simulink model "simulink_p"  (R2018b)
settings: Solver=VariableStepAuto  StartTime=0.0  StopTime=10.0  RelTol=1e-3
undefined symbols (not defined in the file): kp, kp1, td, ti, ti1
settings Model: Creator=tiago  LastModifiedBy=tiago

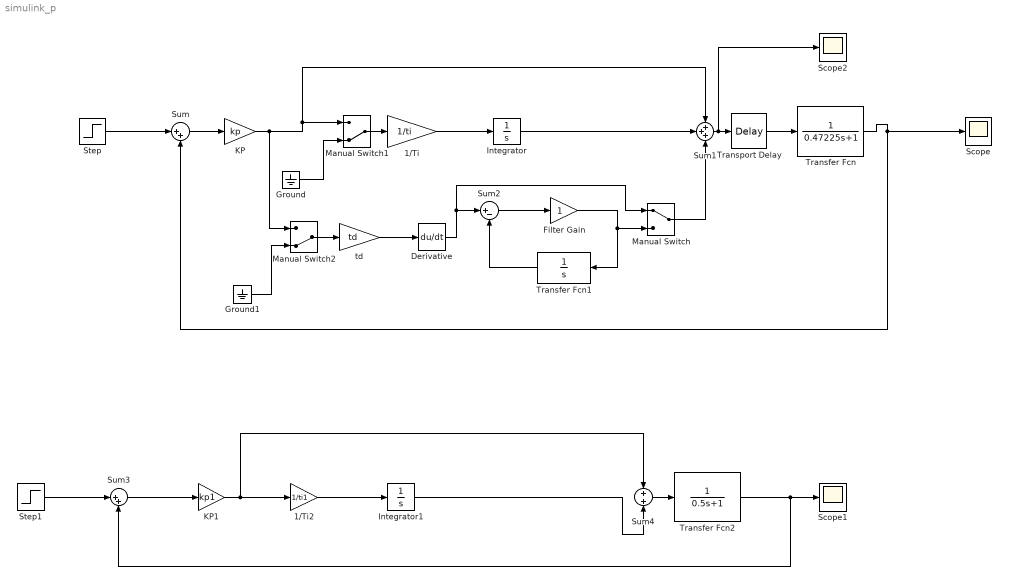
== system simulink_p ==
  1/Ti : Gain  Gain=1/ti
  1/Ti2 : Gain  Gain=1/ti1
  Derivative : Derivative
  Filter Gain : Gain
  Ground : Ground
  Ground1 : Ground
  Integrator : Integrator
  Integrator1 : Integrator
  KP : Gain  Gain=kp
  KP1 : Gain  Gain=kp1
  Manual Switch : ManualSwitch
  Manual Switch1 : ManualSwitch  CurrentSetting=0
  Manual Switch2 : ManualSwitch  CurrentSetting=0
  Scope : Scope
  Scope1 : Scope
  Scope2 : Scope
  Step : Step  Time=0.8  SampleTime=0.3
  Step1 : Step  Time=0.8  SampleTime=2
  Sum : Sum  Inputs=|++
  Sum1 : Sum  Inputs=+++
  Sum2 : Sum  Inputs=|+-
  Sum3 : Sum  Inputs=|++
  Sum4 : Sum
  Transfer Fcn : TransferFcn  Denominator=[0.47225 1]
  Transfer Fcn1 : TransferFcn  Denominator=[1 0]
  Transfer Fcn2 : TransferFcn  Denominator=[0.5 1]
  Transport Delay : TransportDelay
  td : Gain  Gain=td
  wires:
  Step/1 -> Sum/1
  1/Ti/1 -> Integrator/1
  Integrator/1 -> Sum1/2
  KP/1 -> Manual Switch1/1, Sum1/1, Manual Switch2/1
  td/1 -> Derivative/1
  Sum/1 -> KP/1
  Derivative/1 -> Manual Switch/1, Sum2/1
  Transfer Fcn1/1 -> Sum2/2
  Sum2/1 -> Filter Gain/1
  Filter Gain/1 -> Transfer Fcn1/1, Manual Switch/2
  Manual Switch/1 -> Sum1/3
  Transfer Fcn/1 -> Sum/2, Scope/1
  Sum4/1 -> Transfer Fcn2/1
  Step1/1 -> Sum3/1
  KP1/1 -> 1/Ti2/1, Sum4/1
  1/Ti2/1 -> Integrator1/1
  Integrator1/1 -> Sum4/2
  Sum3/1 -> KP1/1
  Transfer Fcn2/1 -> Scope1/1, Sum3/2
  Sum1/1 -> Scope2/1, Transport Delay/1
  Transport Delay/1 -> Transfer Fcn/1
  Manual Switch1/1 -> 1/Ti/1
  Ground/1 -> Manual Switch1/2
  Manual Switch2/1 -> td/1
  Ground1/1 -> Manual Switch2/2
